simulink model "semiAvtiveDamper"  (R2020a)
settings: Solver=ode1  StartTime=0.0  StopTime=Tsim  FixedStep=Ts  RelTol=1e-3
values from neighbouring files (symbols this model uses):
  Ts = 0.1    [stateFcn.m]
undefined symbols (not defined in the file or in its folder): ref, x0
libraries: mympclib x1
settings Model: Creator=kohei  LastModifiedBy=kohei

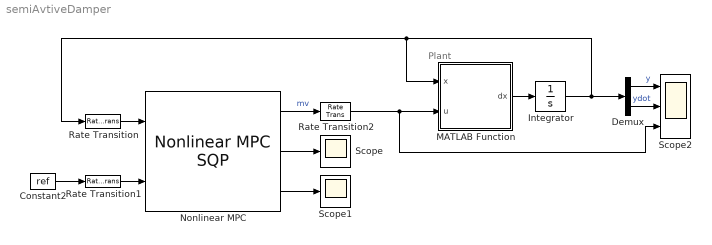
== system semiAvtiveDamper ==
  note: Plant
  Constant2 : Constant  Value=ref
  Demux : Demux  Outputs=2
  Integrator : Integrator  InitialCondition=x0
  MATLAB Function : MATLAB Function  TreatAsAtomicUnit=on
  Nonlinear MPC : mympclib/Nonlinear MPC SQP  params=params  ny=ny  nu=nu  Ts=Ts  enableDist=off  nd=0  enableSlack=on  enableStatus=on
      settings: SourceProductName=My MPC Library
  Rate Transition : RateTransition  InitialCondition=x0
  Rate Transition1 : RateTransition
  Rate Transition2 : RateTransition
  Scope : Scope
  Scope1 : Scope
  Scope2 : Scope  NumInputPorts=3
  wires:
  MATLAB Function/1(dx) -> Integrator/1
  Integrator/1 -> Demux/1, MATLAB Function/1(x), Rate Transition/1
  Nonlinear MPC/2 -> Scope/1
  Nonlinear MPC/3 -> Scope1/1
  Rate Transition/1 -> Nonlinear MPC/1
  Constant2/1 -> Rate Transition1/1
  Rate Transition1/1 -> Nonlinear MPC/2
  Demux/1 -> Scope2/1  "y"
  Demux/2 -> Scope2/2  "ydot"
  Nonlinear MPC/1 -> Rate Transition2/1  "mv"
  Rate Transition2/1 -> Scope2/3, MATLAB Function/2(u)

== matlab function semiAvtiveDamper/MATLAB Function ==
  data: x input; u input; dx output
function dx = fcn(x,u)
m = 2;
k = 1;
dx = [x(2);
     -1/m*(k*x(1)+x(2)*u(1));
     ];
end
